simulink model "car_pend_system_pid_and_lqr_2016a"  (R2016a)
settings: Solver=ode15s  SolverMode=SingleTasking  StartTime=0.0  StopTime=10  MaxStep=0.01  RelTol=1e-3
InitFcn:
  | %系统状态空间描述
  | A = [0	1	          0	         0;
  |      0	-0.166666666666667	1.63333333333333	0;
  |      0	0	          0	         1;
  |      0	-0.277777777777778	19.0555555555556	0];
  | B = [0 1.66666666666667 0 2.77777777777778]';
  | C = [1 0 0 0; 0 0 1 0];
  | D = zeros(2,1);
  | 
  | %全维状态观测器设计
  | foe_p = [-20 -15 -25 -10];
  | L = place(A', C', foe_p);
  | L = L';
  | A_foe = A - L*C;
  | B_foe = [B L];
  | C_foe = eye(4);
  | D_foe = zeros(4,3);
  | 
  | %降维状态观测器设计
  | R = [0 1 1 0; 1 0 0 1];
  | P = [C; R];
  | Q = inv(P);
  | Q1 = Q( : , 1 : 2);
  | Q2 = Q( : , 3 : 4);
  | A_hat = P*A*Q;
  | A11 = A_hat(1:2, 1:2);
  | A12 = A_hat(1:2, 3:4);
  | A21 = A_hat(3:4, 1:2);
  | A22 = A_hat(3:4, 3:4);
  | B_hat = P*B;
  | B1 = B_hat(1:2, : );
  | B2 = B_hat(3:4, : );
  | roe_p = [-18 -20];
  | L_hat = place(A22', A12', roe_p);
  | L_hat = L_hat';
  | A_roe = A22 - L_hat*A12;
  | B_roe1 = A21 - L_hat*A11 + (A22 - L_hat*A12)*L_hat;
  | B_roe2 = B2 - L_hat*B1;
  | B_roe = [B_roe2 B_roe1];
  | C_roe = eye(2);
  | D_roe = zeros(2, 3);
  | y_coef = Q1 + Q2*L_hat;
  | 
  | %全状态反馈极点配置
  | %p = [-2+2i -2-2i -3+2i -3-2i];
  | p = [-4+4i -4-4i -6+3i -6-3i];
  | K_FSFB = place(A, B, p);
  | 
  | %lqr控制器极点配置
  | Q = C'*C;
  | Q(1, 1) = 10;
  | Q(3, 3) = 1000;
  | R = 0.01;
  | K_LQR = lqr(A, B, Q, R);
model workspace (MAT data in the model file):
  car_h = 0.1
  car_l = 0.2
  car_rho = 250
  car_w = 0.1
  pend_h = 0.05
  pend_l = 0.6
  pend_rho = 133.33
  pend_w = 0.05
undefined symbols (not defined in the file): X, Y, Z
libraries: sm_lib x9, nesl_utility x6, simulink x3
settings Model: Creator=sunji  LastModifiedBy=jasper
settings DataIOCC: ReturnWorkspaceOutputs=on
settings DebuggingCC: SFUnexpectedBacktrackingDiag=error  SFNoUnconditionalDefaultTransitionDiag=error
settings SFSimCC: SimUseLocalCustomCode=on
settings RTWCC: RTWUseLocalCustomCode=on
settings GRTTargetCC: TargetLangStandard=C99 (ISO)
settings ConfigComp: CovMetricSettings=dwe  CovSaveCumulativeToWorkspaceVar=off  CovSaveSingleToWorkspaceVar=off  CovExternalEMLEnable=on
settings ExplorerConfigSet: InternalSimMechanicsExplorerSettings="<ExplorerConfiguration><canonicalview>default</canonicalview><AnimationSetting><BasePlaybackSpeed>1.0</BasePlaybackSpeed><PlaybackSpeedFactor>2.0</PlaybackSpeedFactor></AnimationSetting><TilePanel><TileInfo><Tiles Columns=\"1\" Count=\"1\" Rows=\"1\"><Column Weight=\"1\"/><Row Weight=\"1\"/><Tile Height=\"1\" Width=\"1\" X=\"0\" Y=\"0\"/></Tiles></TileInfo><SceneInfo><SceneViewer><BGColor><R>1</R><G>1</G><B>1</B></BGColor><Camera><DoPerspective>off</DoPerspective><Position><X>-0.941380862456283829</X><Y>-8.04082988328747739</Y><Z>0.376092800407251571</Z></Position><Center><X>-0.941380862456283829</X><Y>-5.5511151231257827e-17</Y><Z>0.376092800407251571</Z></Center><Up><X>0</X><Y>-0</Y><Z>1</Z></Up><ViewLimDist>1</ViewLimDist><YLim>1.48375406700784307</YLim><XLim>2.52745317919197099</XLim></Camera></SceneViewer></SceneInfo></TilePanel><MechEditorPanel><Cameras/><GfxPanelCameraMap/><VideoCreator><PlaybackSpeedRatio>1.0</PlaybackSpeedRatio><FrameRate>60</FrameRate><VideoFormat>MPEG-4</VideoFormat><FrameSize>[1280 720]</FrameSize></VideoCreator></MechEditorPanel></ExplorerConfiguration>"

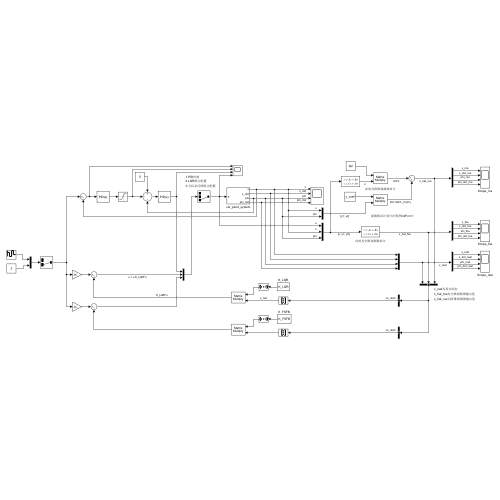
[thumbnail: Simulink's stored preview of the top-level diagram]
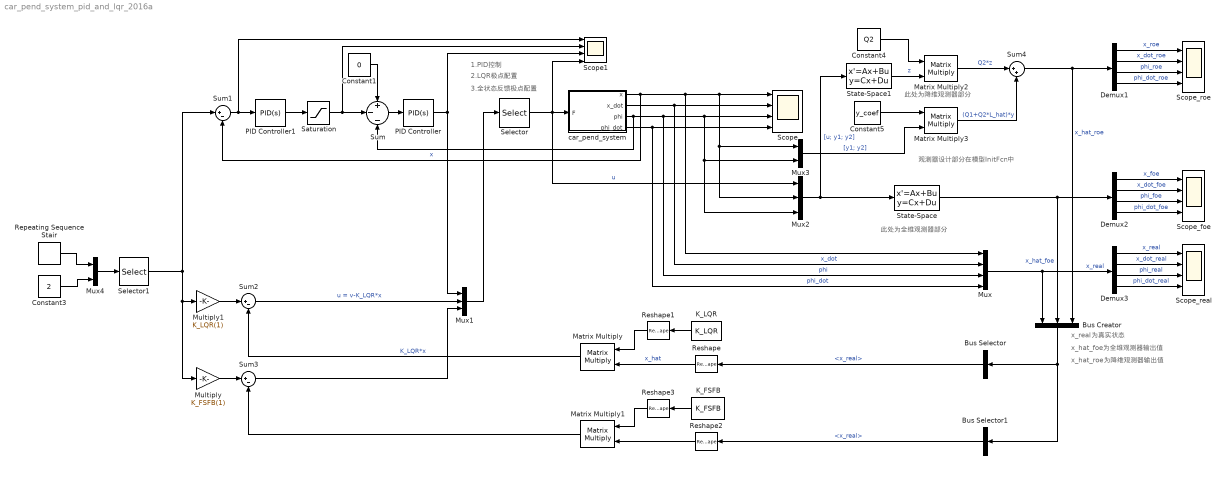
== system car_pend_system_pid_and_lqr_2016a ==
  note: 观测器设计部分在模型InitFcn中
  note: x_hat_roe为降维观测器输出值
  note: x_hat_foe为全维观测器输出值
  note: x_real为真实状态
  note: 3.全状态反馈极点配置
  note: 2.LQR极点配置
  note: 1.PID控制
  note: 此处为降维观测器部分
  note: 此处为全维观测器部分
  Bus Creator : BusCreator  Inputs=3
  Bus Selector : BusSelector  OutputSignals=x_real
  Bus Selector1 : BusSelector  OutputSignals=x_real
  Constant1 : Constant  Value=0
  Constant3 : Constant  Value=2
  Constant4 : Constant  Value=Q2
  Constant5 : Constant  Value=y_coef
  Demux1 : Demux
  Demux2 : Demux
  Demux3 : Demux
  K_FSFB : Constant  Value=K_FSFB
  K_LQR : Constant  Value=K_LQR
  Matrix Multiply{,1..3} (4 alike) : Product  Multiplication=Matrix(*)
  Multiply : Gain  Gain=K_FSFB(1)
  Multiply1 : Gain  Gain=K_LQR(1)
  Mux : Mux
  Mux1 : Mux  Inputs=3
  Mux2 : Mux  Inputs=3
  Mux3 : Mux  Inputs=2
  Mux4 : Mux  Inputs=2
  PID Controller : simulink/Continuous/PID Controller  Controller=PID  Form=Parallel  TimeDomain=Continuous-time  SampleTime=-1  IntegratorMethod=Forward Euler  ControllerParametersSource=internal  P=62.8945166558396  I=123.729251384165  D=6.08832406037103  UseFilter=on  N=3170.92295169654  InitialConditionSource=internal  InitialConditionForIntegrator=0  InitialConditionForFilter=0  DifferentiatorICPrevScaledInput=0  ExternalReset=none  TrackingMode=off  Kt=1  LimitOutput=off  UpperSaturationLimit=inf  LowerSaturationLimit=-inf  LinearizeAsGain=on  AntiWindupMode=none  Kb=1  POutMin=[]  POutMax=[]  IOutMin=[]  IOutMax=[]  DOutMin=[]  DOutMax=[]  NOutMin=[]  NOutMax=[]  SumOutMin=[]  SumOutMax=[]  SaturationOutMin=[]  SaturationOutMax=[]  PParamMin=[]  PParamMax=[]  IParamMin=[]  IParamMax=[]  DParamMin=[]  DParamMax=[]  NParamMin=[]  NParamMax=[]  KbParamMin=[]  KbParamMax=[]  KtParamMin=[]  KtParamMax=[]  KbOutMin=[]  KbOutMax=[]  KtOutMin=[]  KtOutMax=[]  IntegratorOutMin=[]  IntegratorOutMax=[]  FilterOutMin=[]  FilterOutMax=[]  SumI1OutMin=[]  SumI1OutMax=[]  SumI2OutMin=[]  SumI2OutMax=[]  SumI3OutMin=[]  SumI3OutMax=[]  SumDOutMin=[]  SumDOutMax=[]  DifferentiatorOutMin=[]  DifferentiatorOutMax=[]  IntegratorContinuousStateAttributes=''  IntegratorStateMustResolveToSignalObject=off  IntegratorRTWStateStorageClass=Auto  FilterContinuousStateAttributes=''  FilterStateMustResolveToSignalObject=off  FilterRTWStateStorageClass=Auto
  PID Controller1 : simulink/Continuous/PID Controller  Controller=PID  Form=Parallel  TimeDomain=Continuous-time  SampleTime=-1  IntegratorMethod=Forward Euler  ControllerParametersSource=internal  P=0.111330089310441  I=0.00232165519456277  D=0.224164019675191  UseFilter=on  N=2.49376558603491  InitialConditionSource=internal  InitialConditionForIntegrator=0  InitialConditionForFilter=0  DifferentiatorICPrevScaledInput=0  ExternalReset=none  TrackingMode=off  Kt=1  LimitOutput=off  UpperSaturationLimit=inf  LowerSaturationLimit=-inf  LinearizeAsGain=on  AntiWindupMode=none  Kb=1  POutMin=[]  POutMax=[]  IOutMin=[]  IOutMax=[]  DOutMin=[]  DOutMax=[]  NOutMin=[]  NOutMax=[]  SumOutMin=[]  SumOutMax=[]  SaturationOutMin=[]  SaturationOutMax=[]  PParamMin=[]  PParamMax=[]  IParamMin=[]  IParamMax=[]  DParamMin=[]  DParamMax=[]  NParamMin=[]  NParamMax=[]  KbParamMin=[]  KbParamMax=[]  KtParamMin=[]  KtParamMax=[]  KbOutMin=[]  KbOutMax=[]  KtOutMin=[]  KtOutMax=[]  IntegratorOutMin=[]  IntegratorOutMax=[]  FilterOutMin=[]  FilterOutMax=[]  SumI1OutMin=[]  SumI1OutMax=[]  SumI2OutMin=[]  SumI2OutMax=[]  SumI3OutMin=[]  SumI3OutMax=[]  SumDOutMin=[]  SumDOutMax=[]  DifferentiatorOutMin=[]  DifferentiatorOutMax=[]  IntegratorContinuousStateAttributes=''  IntegratorStateMustResolveToSignalObject=off  IntegratorRTWStateStorageClass=Auto  FilterContinuousStateAttributes=''  FilterStateMustResolveToSignalObject=off  FilterRTWStateStorageClass=Auto
  Repeating Sequence Stair : simulink/Sources/Repeating Sequence Stair  OutValues=[3 1 4 2].'  tsamp=5  OutMin=[]  OutMax=[]  OutDataTypeStr=double  OutputDataTypeScalingMode=double  OutDataType=fixdt(0,8)  ConRadixGroup=Best Precision: Vector-wise  OutScaling=2^-12
  Reshape : Reshape  OutputDimensionality=Column vector (2-D)
  Reshape1 : Reshape  OutputDimensionality=Row vector (2-D)
  Reshape2 : Reshape  OutputDimensionality=Column vector (2-D)
  Reshape3 : Reshape  OutputDimensionality=Row vector (2-D)
  Saturation : Saturate  UpperLimit=pi/4  LowerLimit=-pi/4
  Scope : Scope  NumInputPorts=4
  Scope1 : Scope  NumInputPorts=4
  Scope_foe : Scope  NumInputPorts=4
  Scope_real : Scope  NumInputPorts=4
  Scope_roe : Scope  NumInputPorts=4
  Selector : Selector  InputPortWidth=3  IndexOptions=Index vector (dialog)  Indices=[3]  OutputSizes=1
  Selector1 : Selector  InputPortWidth=2  IndexOptions=Index vector (dialog)  Indices=[2]  OutputSizes=1
  State-Space : StateSpace  A=A_foe  B=B_foe  C=C_foe  D=D_foe  X0=0
  State-Space1 : StateSpace  A=A_roe  B=B_roe  C=C_roe  D=D_roe  X0=0
  Sum : Sum  Inputs=+|-|-
  Sum1 : Sum  Inputs=|+-
  Sum2 : Sum  Inputs=|+-
  Sum3 : Sum  Inputs=|+-
  Sum4 : Sum  Inputs=|++
  car_pend_system : Subsystem
  wires:
  car_pend_system/2(x_dot) -> Mux/2, Scope/2  "x_dot"
  car_pend_system/3(phi) -> Sum/3, Mux/3, Scope/3, Mux3/2, Mux2/3  "phi"
  car_pend_system/4(phi_dot) -> Scope/4, Mux/4  "phi_dot"
  car_pend_system/1(x) -> Sum1/2, Mux/1, Mux3/1, Mux2/2, Scope/1  "x"
  Sum1/1 -> PID Controller1/1, Scope1/1
  Saturation/1 -> Sum/2, Scope1/2
  Sum/1 -> PID Controller/1
  PID Controller1/1 -> Saturation/1
  K_LQR/1 -> Reshape1/1
  Reshape1/1 -> Matrix Multiply/1
  Reshape/1 -> Matrix Multiply/2  "x_hat"
  Matrix Multiply/1 -> Sum2/2  "K_LQR*x"
  PID Controller/1 -> Scope1/3, Mux1/1
  Sum2/1 -> Mux1/2  "u = v-K_LQR*x"
  Mux1/1 -> Selector/1
  Selector/1 -> Scope1/4, Mux2/1, car_pend_system/1(F)  "u"
  Constant1/1 -> Sum/1
  Reshape2/1 -> Matrix Multiply1/2
  Reshape3/1 -> Matrix Multiply1/1
  K_FSFB/1 -> Reshape3/1
  Matrix Multiply1/1 -> Sum3/2
  Sum3/1 -> Mux1/3
  Mux2/1 -> State-Space1/1, State-Space/1  "[u; y1; y2]"
  State-Space/1 -> Bus Creator/2, Demux2/1  "x_hat_foe"
  State-Space1/1 -> Matrix Multiply2/2  "z"
  Constant4/1 -> Matrix Multiply2/1
  Matrix Multiply2/1 -> Sum4/1  "Q2*z"
  Constant5/1 -> Matrix Multiply3/1
  Mux3/1 -> Matrix Multiply3/2  "[y1; y2]"
  Matrix Multiply3/1 -> Sum4/2  "(Q1+Q2*L_hat)*y"
  Sum4/1 -> Demux1/1, Bus Creator/3  "x_hat_roe"
  Demux1/1 -> Scope_roe/1  "x_roe"
  Demux1/2 -> Scope_roe/2  "x_dot_roe"
  Demux1/3 -> Scope_roe/3  "phi_roe"
  Demux1/4 -> Scope_roe/4  "phi_dot_roe"
  Demux2/3 -> Scope_foe/3  "phi_foe"
  Demux2/2 -> Scope_foe/2  "x_dot_foe"
  Demux2/4 -> Scope_foe/4  "phi_dot_foe"
  Demux2/1 -> Scope_foe/1  "x_foe"
  Demux3/4 -> Scope_real/4  "phi_dot_real"
  Demux3/3 -> Scope_real/3  "phi_real"
  Mux/1 -> Bus Creator/1, Demux3/1  "x_real"
  Demux3/2 -> Scope_real/2  "x_dot_real"
  Demux3/1 -> Scope_real/1  "x_real"
  Multiply/1 -> Sum3/1
  Multiply1/1 -> Sum2/1
  Bus Creator/1 -> Bus Selector1/1, Bus Selector/1
  Bus Selector/1 -> Reshape/1  "<x_real>"
  Bus Selector1/1 -> Reshape2/1  "<x_real>"
  Constant3/1 -> Mux4/2
  Repeating Sequence Stair/1 -> Mux4/1
  Mux4/1 -> Selector1/1
  Selector1/1 -> Multiply/1, Multiply1/1, Sum1/1

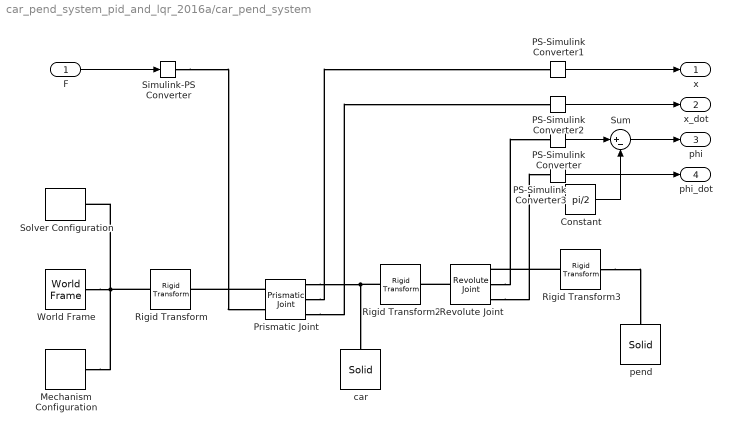
== system car_pend_system_pid_and_lqr_2016a/car_pend_system ==
  F : Inport
  Constant : Constant  Value=pi/2
  Mechanism Configuration : sm_lib/Utilities/Mechanism Configuration  UniformGravity=Constant  GravityVector=[0 0 -9.8]  GravityUnits=m/s^2  LinearizationDelta=0.001  JointModeTransitionNonlinearIterations=2
  PS-Simulink Converter{,1..3} (4 alike) : nesl_utility/PS-Simulink Converter  PhysicalDomain=network_engine_domain  SubClassName=ps_output  LeftPortType=input  RightPortType=output  PseudoPeriodic=off  Frequencies=[]  Unit=inherit  AffineConversion=off
  Prismatic Joint : sm_lib/Joints/Prismatic Joint  JointMode=Normal  SenseConstraintForce=off  SenseConstraintForceX=off  SenseConstraintForceY=off  SenseConstraintForceZ=off  SenseConstraintTorque=off  SenseConstraintTorqueX=off  SenseConstraintTorqueY=off  SenseConstraintTorqueZ=off  SenseTotalForce=off  SenseTotalForceX=off  SenseTotalForceY=off  SenseTotalForceZ=off  SenseTotalTorque=off  SenseTotalTorqueX=off  SenseTotalTorqueY=off  SenseTotalTorqueZ=off  CompositeWrenchDir=FollowerOnBase  CompositeWrenchFrame=BaseFrame  EquilibriumPosition=0  EquilibriumPositionUnits=m  SpringStiffness=0  SpringStiffnessUnits=N/m  DampingCoefficient=0.1  DampingCoefficientUnits=N/(m/s)  TorqueActuationMode=InputTorque  MotionActuationMode=ComputedMotion  SensePosition=on  SenseVelocity=on  SenseAcceleration=off  SenseTorqueForce=off  SenseLowerLimitTorqueForce=off  SenseUpperLimitTorqueForce=off  LowerLimitSpecify=off  LowerLimitBound=-1  LowerLimitBoundUnits=m  LowerLimitStiffness=1e6  LowerLimitStiffnessUnits=N/m  LowerLimitDamping=1e3  LowerLimitDampingUnits=N/(m/s)  LowerLimitTransitionRegionWidth=1e-4  LowerLimitTransitionRegionWidthUnits=m  UpperLimitSpecify=off  UpperLimitBound=1  UpperLimitBoundUnits=m  UpperLimitStiffness=1e6  UpperLimitStiffnessUnits=N/m  UpperLimitDamping=1e3  UpperLimitDampingUnits=N/(m/s)  UpperLimitTransitionRegionWidth=1e-4  UpperLimitTransitionRegionWidthUnits=m  PositionTargetSpecify=off  PositionTargetPriority=High  PositionTargetValue=0  PositionTargetValueUnits=m  VelocityTargetSpecify=off  VelocityTargetPriority=High  VelocityTargetValue=0  VelocityTargetValueUnits=m/s
  Revolute Joint : sm_lib/Joints/Revolute Joint  JointMode=Normal  SenseConstraintForce=off  SenseConstraintForceX=off  SenseConstraintForceY=off  SenseConstraintForceZ=off  SenseConstraintTorque=off  SenseConstraintTorqueX=off  SenseConstraintTorqueY=off  SenseConstraintTorqueZ=off  SenseTotalForce=off  SenseTotalForceX=off  SenseTotalForceY=off  SenseTotalForceZ=off  SenseTotalTorque=off  SenseTotalTorqueX=off  SenseTotalTorqueY=off  SenseTotalTorqueZ=off  CompositeWrenchDir=FollowerOnBase  CompositeWrenchFrame=BaseFrame  EquilibriumPosition=0  EquilibriumPositionUnits=deg  SpringStiffness=0  SpringStiffnessUnits=N*m/deg  DampingCoefficient=0  DampingCoefficientUnits=N*m/(deg/s)  TorqueActuationMode=NoTorque  MotionActuationMode=ComputedMotion  SensePosition=on  SenseVelocity=on  SenseAcceleration=off  SenseTorqueForce=off  SenseLowerLimitTorqueForce=off  SenseUpperLimitTorqueForce=off  LowerLimitSpecify=off  LowerLimitBound=-90  LowerLimitBoundUnits=deg  LowerLimitStiffness=0  LowerLimitStiffnessUnits=N*m/deg  LowerLimitDamping=0  LowerLimitDampingUnits=N*m/(deg/s)  LowerLimitTransitionRegionWidth=0.1  LowerLimitTransitionRegionWidthUnits=deg  UpperLimitSpecify=off  UpperLimitBound=90  UpperLimitBoundUnits=deg  UpperLimitStiffness=0  UpperLimitStiffnessUnits=N*m/deg  UpperLimitDamping=0  UpperLimitDampingUnits=N*m/(deg/s)  UpperLimitTransitionRegionWidth=0.1  UpperLimitTransitionRegionWidthUnits=deg  PositionTargetSpecify=on  PositionTargetPriority=Low  PositionTargetValue=90  PositionTargetValueUnits=deg  VelocityTargetSpecify=off  VelocityTargetPriority=Low  VelocityTargetValue=5  VelocityTargetValueUnits=deg/s
  Rigid Transform : sm_lib/Frames and Transforms/Rigid Transform  TranslationMethod=StandardAxis  TranslationStandardOffset=car_h/2  TranslationLengthUnit=m  TranslationStandardAxis=+Z  TranslationCartesianOffset=[0 0 0]  TranslationROffset=0  TranslationROffsetUnits=m  TranslationZOffset=0  TranslationZOffsetUnits=m  TranslationThetaOffset=0  TranslationThetaOffsetUnits=deg  RotationMethod=StandardAxis  RotationAngleUnits=deg  RotationStandardAxis=+Y  RotationAngle=90.0  RotationArbitraryAxis=[0 0 1]  FollAlignAxisA=+X  BaseAlignAxisA=+Y  FollAlignAxisB=+Y  BaseAlignAxisB=+Z  RotationSequenceAxes=FollowerAxes  RotationSequence=XYX  RotationSequenceAngles=[0 0 0]  RotationSequenceAnglesUnits=deg  RotationMatrix=[1 0 0; 0 1 0; 0 0 1]
  Rigid Transform2 : sm_lib/Frames and Transforms/Rigid Transform  TranslationMethod=None  TranslationStandardOffset=car_h/2  TranslationLengthUnit=m  TranslationStandardAxis=-X  TranslationCartesianOffset=[0 0 0]  TranslationROffset=0  TranslationROffsetUnits=m  TranslationZOffset=0  TranslationZOffsetUnits=m  TranslationThetaOffset=0  TranslationThetaOffsetUnits=deg  RotationMethod=StandardAxis  RotationAngleUnits=deg  RotationStandardAxis=+X  RotationAngle=90.0  RotationArbitraryAxis=[0 0 1]  FollAlignAxisA=+X  BaseAlignAxisA=+Y  FollAlignAxisB=+Y  BaseAlignAxisB=+Z  RotationSequenceAxes=FollowerAxes  RotationSequence=XYX  RotationSequenceAngles=[0 0 0]  RotationSequenceAnglesUnits=deg  RotationMatrix=[1 0 0; 0 1 0; 0 0 1]
  Rigid Transform3 : sm_lib/Frames and Transforms/Rigid Transform  TranslationMethod=StandardAxis  TranslationStandardOffset=pend_l/2  TranslationLengthUnit=m  TranslationStandardAxis=+Y  TranslationCartesianOffset=[0 0 0]  TranslationROffset=0  TranslationROffsetUnits=m  TranslationZOffset=0  TranslationZOffsetUnits=m  TranslationThetaOffset=0  TranslationThetaOffsetUnits=deg  RotationMethod=StandardAxis  RotationAngleUnits=deg  RotationStandardAxis=+Z  RotationAngle=90.0  RotationArbitraryAxis=[0 0 1]  FollAlignAxisA=+X  BaseAlignAxisA=+Y  FollAlignAxisB=+Y  BaseAlignAxisB=+Z  RotationSequenceAxes=FollowerAxes  RotationSequence=XYX  RotationSequenceAngles=[0 0 0]  RotationSequenceAnglesUnits=deg  RotationMatrix=[1 0 0; 0 1 0; 0 0 1]
  Simulink-PS Converter : nesl_utility/Simulink-PS Converter  PhysicalDomain=network_engine_domain  SubClassName=ps_input  LeftPortType=input  RightPortType=output  PseudoPeriodic=off  Frequencies=[]  NoiseDistribution=none  NoiseParameters=[]  Unit=1  AffineConversion=off  FilteringAndDerivatives=provide  SimscapeFilterOrder=1  InputFilterTimeConstant=0.001  UdotUserProvided=0
  Solver Configuration : nesl_utility/Solver Configuration  PhysicalDomain=network_engine_domain  SubClassName=solver  LeftPortType=input  RightPortType=generic  Tones=[]  Harmonics=[]  SimulateNoise=off  Profile=off  UseLocalSampling=off  EnableSwitchedLinearOptims=on  FrequencyDomain=off  UseCCode=off  RelTol=0.001  AbsTol=1e-06  MinStep=1e-09  ToWorkspace=off  RevertToSquareIcSolve=off  NumHomotopyIterations=100  PhasorMode=off  PhasorModeNumHarmonics=1  DoDC=off  ResidualTolerance=1e-09  UseLocalSolver=off  LocalSolverChoice=NE_BACKWARD_EULER_ADVANCER  LocalSolverSampleTime=0.001  DoFixedCost=off  MaxNonlinIter=3  MaxModeIter=2  ComputeImpulses=off  ImpulseIterations=2  LinearAlgebra=Sparse  EquationFormulation=NE_TIME_EF  DelaysMemoryBudget=1024  AutomaticFiltering=on  FilteringTimeConstant=0.001  PartitionStorageMethod=AS_NEEDED  PartitionMemoryBudget=1024  PartitionMethod=FAST
  Sum : Sum  Inputs=|+-
  World Frame : sm_lib/Frames and Transforms/World Frame
  car : sm_lib/Body Elements/Solid  GraphicAmbientColor=[0.15 0.15 0.15 1.0]  BasedOnType=Density  BrickDimensions=[car_h car_w car_l]  BrickDimensionUnits=m  CenterOfMass=[0 0 0]  CenterOfMassUnits=m  GraphicDiffuseColor=[0.6 0.6 0.6]  Density=car_rho  DensityUnits=kg/m^3  DoExposeReferenceFrame=on  GraphicEmissiveColor=[0.0 0.0 0.0 1.0]  ExportEntireGeometry=off  SerializedFrames=<Frames/>  MarkerShape=Sphere  MarkerSize=10  GraphicType=FromGeometry  InertiaType=CalculateFromGeometry  Mass=1  MassUnits=kg  MomentsOfInertia=[1 1 1]  MomentsOfInertiaUnits=kg*m^2  GraphicOpacity=1.0  ProductsOfInertia=[0 0 0]  ProductsOfInertiaUnits=kg*m^2  GraphicShininess=75  GraphicSpecularColor=[0.5 0.5 0.5 1.0]  GraphicVisPropType=SimpleVisualProperties  GeometryShape=Brick
  pend : sm_lib/Body Elements/Solid  GraphicAmbientColor=[0.15 0.15 0.15 1.0]  BasedOnType=Density  BrickDimensions=[pend_l pend_w pend_h]  BrickDimensionUnits=m  CenterOfMass=[0 0 0]  CenterOfMassUnits=m  GraphicDiffuseColor=[0.6 0.0 0.2]  Density=pend_rho  DensityUnits=kg/m^3  DoExposeReferenceFrame=on  GraphicEmissiveColor=[0.0 0.0 0.0 1.0]  ExportEntireGeometry=off  SerializedFrames=<Frames/>  MarkerShape=Sphere  MarkerSize=10  GraphicType=FromGeometry  InertiaType=CalculateFromGeometry  Mass=1  MassUnits=kg  MomentsOfInertia=[1 1 1]  MomentsOfInertiaUnits=kg*m^2  GraphicOpacity=1.0  ProductsOfInertia=[0 0 0]  ProductsOfInertiaUnits=kg*m^2  GraphicShininess=75  GraphicSpecularColor=[0.5 0.5 0.5 1.0]  GraphicVisPropType=SimpleVisualProperties  GeometryShape=Brick
  x : Outport
  x_dot : Outport  Port=2
  phi : Outport  Port=3
  phi_dot : Outport  Port=4
  wires:
  F/1 -> Simulink-PS Converter/1
  PS-Simulink Converter1/1 -> x/1
  PS-Simulink Converter3/1 -> phi_dot/1
  PS-Simulink Converter2/1 -> x_dot/1
  PS-Simulink Converter/1 -> Sum/1
  Sum/1 -> phi/1
  Constant/1 -> Sum/2
  connections:
  Revolute Joint/LConn1 -- Rigid Transform2/RConn1
  Revolute Joint/RConn2 -- PS-Simulink Converter/LConn1
  World Frame/RConn1 -- Rigid Transform/LConn1 -- Solver Configuration/RConn1 -- Mechanism Configuration/RConn1
  Prismatic Joint/RConn2 -- PS-Simulink Converter1/LConn1
  Revolute Joint/RConn3 -- PS-Simulink Converter3/LConn1
  Prismatic Joint/RConn3 -- PS-Simulink Converter2/LConn1
  Rigid Transform3/LConn1 -- Revolute Joint/RConn1
  Prismatic Joint/RConn1 -- Rigid Transform2/LConn1 -- car/RConn1
  Simulink-PS Converter/RConn1 -- Prismatic Joint/LConn2
  Rigid Transform3/RConn1 -- pend/RConn1
  Prismatic Joint/LConn1 -- Rigid Transform/RConn1
